simulink model "Problem1"  (R2017a)
settings: Solver=ode23  StartTime=0.0  StopTime=0.5  MaxStep=0.001  MinStep=0.0001  RelTol=1e-5
undefined symbols (not defined in the file): C, L, R
settings Model: Creator=Gowtham  LastModifiedBy=Gowtham

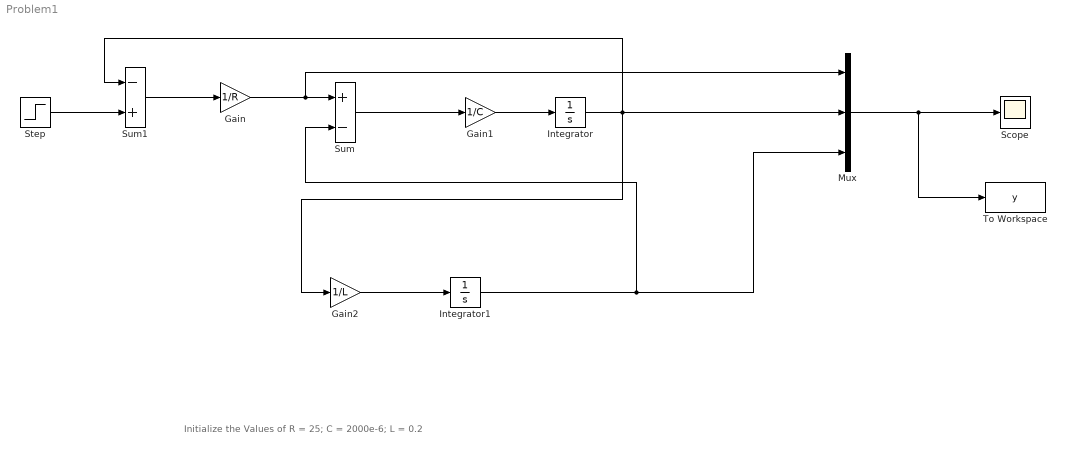
== system Problem1 ==
  note: Initialize the Values of R = 25; C = 2000e-6; L = 0.2
  Gain : Gain  Gain=1/R
  Gain1 : Gain  Gain=1/C
  Gain2 : Gain  Gain=1/L
  Integrator : Integrator
  Integrator1 : Integrator
  Mux : Mux  Inputs=3
  Scope : Scope
  Step : Step  Time=0.01  After=110  SampleTime=0
  Sum : Sum  Inputs=+-
  Sum1 : Sum  Inputs=-+
  To Workspace : ToWorkspace  VariableName=y  SaveFormat=Timeseries  SampleTime=-1
  wires:
  Step/1 -> Sum1/2
  Sum1/1 -> Gain/1
  Gain/1 -> Mux/1, Sum/1
  Sum/1 -> Gain1/1
  Gain1/1 -> Integrator/1
  Integrator/1 -> Mux/2, Sum1/1, Gain2/1
  Gain2/1 -> Integrator1/1
  Integrator1/1 -> Mux/3, Sum/2
  Mux/1 -> To Workspace/1, Scope/1
